simulink model "FuncVisualisation"  (Simulink 7.5)
settings: Solver=ode45  StartTime=0.0  StopTime=100  RelTol=1e-3
undefined symbols (not defined in the file or in its folder): TaylorApproximation, x
libraries: simulink x2
settings Model: Creator=alexcftrk  LastModifiedBy=knifewounded

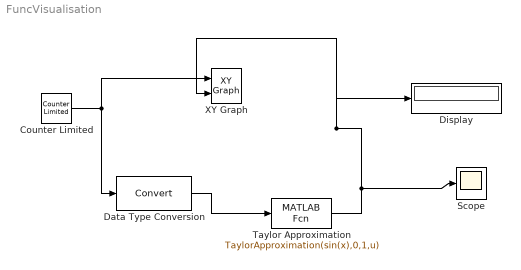
== system FuncVisualisation ==
  Counter Limited : simulink/Sources/Counter Limited  SystemSampleTime=-1  uplimit=10000  tsamp=-1
  Data Type Conversion : DataTypeConversion  OutDataType=fixdt(1, 16)  OutScaling=2^0  ConvertRealWorld=Stored Integer (SI)  RndMeth=Nearest
  Display : Display
  Scope : Scope
  Taylor Approximation : MATLABFcn  MATLABFcn=TaylorApproximation(sin(x),0,1,u)
  XY Graph : simulink/Sinks/XY Graph  SystemSampleTime=-1  xmin=-1  xmax=10  ymin=-1  ymax=10  st=-1
  wires:
  Taylor Approximation/1 -> Scope/1, Display/1, XY Graph/2
  Counter Limited/1 -> Data Type Conversion/1, XY Graph/1
  Data Type Conversion/1 -> Taylor Approximation/1
